simulink model "isubsystem_main"  (R2014b)
settings: Solver=ode45  StartTime=0.0  StopTime=5  FixedStep=0.001  RelTol=1e-3
undefined symbols (not defined in the file): v1, v10, v11, v12, v13, v14, v15, v16, v17, v18, v19, v2, v20, v21, v22, v3, v4, v5, v6, v7, v8, v9
(part 2 of 2)

== matlab function isubsystem_main/Subsystem/reduced-order dynamic gain observer/MATLAB Function ==
  data: lambda2 input; u input; dlambda2 output; yF input; k2 input; L input; dL input; x2_e output
function [dlambda2,x2_e]= fcn(lambda2,u,yF,k2,L,dL)
%#codegen

x2_e = lambda2 + k2*L*yF;
f1_yF = yF;f2_e = yF*x2_e;
dlambda2 = u + f2_e - k2*L*(x2_e + f1_yF)-k2*dL*yF;

== matlab function isubsystem_main/Subsystem/Fuzzy/MATLAB Function ==
  data: W input; yF input; Xi output; dW output; z1 input; Psi input; eta1 input
function [Xi,dW]= fcn(W,yF,z1,Psi,eta1)
%#codegen

Xi = [exp(-0.5*(yF - 8)^2);exp(-0.5*(yF - 4)^2);exp(-0.5*yF^2);exp(-0.5*(yF + 4)^2);exp(-0.5*(yF + 8)^2)];
dW = Psi*z1*Xi - eta1*Psi*W;

== matlab function isubsystem_main/Subsystem/reduced-order dynamic gain observer/Subsystem/MATLAB Function2 ==
  data: L input; yF input; dL output; sigma input; theta input; K input; P input; lP input; epsilon1 input; epsilon2 input; epsilon10 input; epsilon20 input; vartheta input
function dL = fcn(L,yF,sigma,theta,K,P,lP,epsilon1,epsilon2,epsilon10,epsilon20,vartheta)
%#codegen

hphou = 1 + 2*(yF)^2 + 2*(vartheta)^2;
a = (-theta + K)/sigma;
b = (norm(P,2)*epsilon1^2)/(lP*sigma) + ((2*epsilon10^2)^(-1)+(2*epsilon20^2)^(-1))/(lP*sigma);
c = (2*(2 + epsilon2^2)*norm(P,2)*(hphou)/(lP*sigma));
%dL = L/sigma*(-theta*L + norm(P,2)*epsilon1^2/lP + ((2*epsilon10^2)^(-1)+(2*epsilon20^2)^(-1))/lP + norm(P,2)*(epsilon2^4 + phou^2)/(lP*epsilon2^2) + K*L);
dL = a*L^2 + b*L + c*L;

== matlab function isubsystem_main/Subsystem/PPF /MATLAB Function ==
  data: psi0 input; psi output; dpsi output; psiinf input; T input; q input; t input; ddpsi output
function [psi,dpsi,ddpsi]= fcn(psi0,psiinf,T,q,t)
%#codegen
if t >= T
    r = 0;
    dr = 0;
    ddr = 0;
else
    r = (1 - T^(-1)*t)^(q+1)*(cos(3*t))^2;
    dr = -(cos(3*t)*(1 - t/T)^q*(cos(3*t) + q*cos(3*t) - 6*t*sin(3*t) + 6*T*sin(3*t)))/T;
    ddr = 18*sin(3*t)^2*(1 - t/T)^(q + 1) - 18*cos(3*t)^2*(1 - t/T)^(q + 1) + (q*cos(3*t)^2*(q + 1)*(1 - t/T)^(q - 1))/T^2 + (12*cos(3*t)*sin(3*t)*(q + 1)*(1 - t/T)^q)/T;
end
psi = (psi0 - psiinf)*r + psiinf;
dpsi = (psi0 - psiinf)*dr;
ddpsi = (psi0 - psiinf)*ddr;

== matlab function isubsystem_main/Subsystem/Controller1/Subsystem1/MATLAB Function2 ==
  data: dalpha1_dt input; dalpha1_dW input; dalpha1_dL input; dalpha1_dyF input; alpha1 input; yF input; lambda2 input; alpha2 output; dW input; dL input; L input; k2 input; gamma2 input; sigma input; epsilon20 input; epsilon11 input; epsilon22 input; epsilon23 input; epsilon24 input; epsilon25 input; z2 output
function [alpha2,z2] = fcn(dalpha1_dt,dalpha1_dW,dalpha1_dL,dalpha1_dyF,alpha1,yF,lambda2,dW,dL,L,k2,gamma2,sigma,epsilon20,epsilon11,epsilon22,epsilon23,epsilon24,epsilon25)
%#codegen

z2 = lambda2 - alpha1;
x2_e = lambda2 + k2*L*yF;
f1_yF = yF;f2_e = yF*x2_e;
alpha2 = f2_e - k2*L*(x2_e + f1_yF) - k2*dL*yF - dW'*dalpha1_dW - dalpha1_dL*dL - dalpha1_dt - dalpha1_dyF*(x2_e + f1_yF) + 0.5*z2*dalpha1_dyF^2*((epsilon20*L^sigma)^2 + epsilon22^2 + epsilon23^2 + epsilon25^2) + epsilon24^2*z2 + z2/(2*epsilon11^2) + gamma2*z2;

== matlab function isubsystem_main/Subsystem/Controller1/Subsystem2/MATLAB Function ==
  data: alpha2 input; v output; alpha1 input; lambda2 input; l1 input; l2 input; w input
function v = fcn(alpha2,alpha1,lambda2,l1,l2,w)
%#codegen
delta = 0.5;la = 1 - delta;
z2 = lambda2 - alpha1;
zetad = sqrt(z2^2*alpha2^2 + w^2);
%zetal = sqrt(z2^2*l2^2 + (1 - l1)^2*w^2);
zetal = sqrt(z2^2*l2^2 + w^2);
%v = -(1 + l1)*z2*(alpha2^2/zetad + l2^2/((1 - l1)*zetal));
v = -la^(-1)*z2*(alpha2^2/zetad + l2^2/(zetal));

== matlab function isubsystem_main/Subsystem/Controller1/Subsystem/MATLAB Function1 ==
  data: yF input; dalpha1_dt output; psi input; dpsi input; ddpsi input; L input; W input; Xi input; k2 input; b_low input; b_high input; li input; eta0 input; sigma input; gamma1 input; epsilon10 input; epsilon11 input; epsilon12 input; epsilon13 input; epsilon14 input; epsilon15 input; dalpha1_dW output; dalpha1_dL output; dalpha1_dyF output
function [dalpha1_dt,dalpha1_dW,dalpha1_dL,dalpha1_dyF]= fcn(yF,psi,dpsi,ddpsi,L,W,Xi,k2,b_low,b_high,li,eta0,sigma,gamma1,epsilon10,epsilon11,epsilon12,epsilon13,epsilon14,epsilon15)
%#codegen
dalpha1_dt = (yF*dpsi*(li^2 + yF^2)*(eta0 + 2*gamma1))/(2*li^2*psi^2) - (2*yF^3*dpsi*(b_high - yF/(psi*(li^2 + yF^2)^(1/2)))*(b_low + yF/(psi*(li^2 + yF^2)^(1/2)))*((li^4*(b_high*b_low + yF^2/(psi^2*(li^2 + yF^2)))^2*(epsilon11^2 + epsilon12^2 + epsilon13^2 + epsilon15^2))/(2*(li^2 + yF^2)^3*(b_high - yF/(psi*(li^2 + yF^2)^(1/2)))^4*(b_low + yF/(psi*(li^2 + yF^2)^(1/2)))^4) + (L^(2*sigma)*epsilon10^2*li^4*(b_high*b_low + yF^2/(psi^2*(li^2 + yF^2)))^2)/(2*(li^2 + yF^2)^3*(b_high - yF/(psi*(li^2 + yF^2)^(1/2)))^4*(b_low + yF/(psi*(li^2 + yF^2)^(1/2)))^4) + (epsilon14^2*yF^2*dpsi^2*(b_high*b_low + yF^2/(psi^2*(li^2 + yF^2)))^2)/(2*psi^4*(li^2 + yF^2)*(b_high - yF/(psi*(li^2 + yF^2)^(1/2)))^4*(b_low + yF/(psi*(li^2 + yF^2)^(1/2)))^4)))/(li^2*psi^4*(b_high*b_low + yF^2/(psi^2*(li^2 + yF^2)))^2) + (yF*(li^2 + yF^2)*(b_high - yF/(psi*(li^2 + yF^2)^(1/2)))*(b_low + yF/(psi*(li^2 + yF^2)^(1/2)))*((2*epsilon14^2*yF^2*dpsi*dpsi^2*(b_high*b_low + yF^2/(psi^2*(li^2 + yF^2)))^2)/(psi^5*(li^2 + yF^2)*(b_high - yF/(psi*(li^2 + yF^2)^(1/2)))^4*(b_low + yF/(psi*(li^2 + yF^2)^(1/2)))^4) - (2*epsilon14^2*yF^3*dpsi*dpsi^2*(b_high*b_low + yF^2/(psi^2*(li^2 + yF^2)))^2)/(psi^6*(li^2 + yF^2)^(3/2)*(b_high - yF/(psi*(li^2 + yF^2)^(1/2)))^4*(b_low + yF/(psi*(li^2 + yF^2)^(1/2)))^5) + (2*epsilon14^2*yF^3*dpsi*dpsi^2*(b_high*b_low + yF^2/(psi^2*(li^2 + yF^2)))^2)/(psi^6*(li^2 + yF^2)^(3/2)*(b_high - yF/(psi*(li^2 + yF^2)^(1/2)))^5*(b_low + yF/(psi*(li^2 + yF^2)^(1/2)))^4) - (epsilon14^2*yF^2*ddpsi*dpsi*(b_high*b_low + yF^2/(psi^2*(li^2 + yF^2)))^2)/(psi^4*(li^2 + yF^2)*(b_high - yF/(psi*(li^2 + yF^2)^(1/2)))^4*(b_low + yF/(psi*(li^2 + yF^2)^(1/2)))^4) + (2*epsilon14^2*yF^4*dpsi*dpsi^2*(b_high*b_low + yF^2/(psi^2*(li^2 + yF^2))))/(psi^7*(li^2 + yF^2)^2*(b_high - yF/(psi*(li^2 + yF^2)^(1/2)))^4*(b_low + yF/(psi*(li^2 + yF^2)^(1/2)))^4) + (2*li^4*yF^2*dpsi*(b_high*b_low + yF^2/(psi^2*(li^2 + yF^2)))*(epsilon11^2 + epsilon12^2 + epsilon13^2 + epsilon15^2))/(psi^3*(li^2 + yF^2)^4*(b_high - yF/(psi*(li^2 + yF^2)^(1/2)))^4*(b_low + yF/(psi*(li^2 + yF^2)^(1/2)))^4) - (2*li^4*yF*dpsi*(b_high*b_low + yF^2/(psi^2*(li^2 + yF^2)))^2*(epsilon11^2 + epsilon12^2 + epsilon13^2 + epsilon15^2))/(psi^2*(li^2 + yF^2)^(7/2)*(b_high - yF/(psi*(li^2 + yF^2)^(1/2)))^4*(b_low + yF/(psi*(li^2 + yF^2)^(1/2)))^5) + (2*li^4*yF*dpsi*(b_high*b_low + yF^2/(psi^2*(li^2 + yF^2)))^2*(epsilon11^2 + epsilon12^2 + epsilon13^2 + epsilon15^2))/(psi^2*(li^2 + yF^2)^(7/2)*(b_high - yF/(psi*(li^2 + yF^2)^(1/2)))^5*(b_low + yF/(psi*(li^2 + yF^2)^(1/2)))^4) + (2*L^(2*sigma)*epsilon10^2*li^4*yF^2*dpsi*(b_high*b_low + yF^2/(psi^2*(li^2 + yF^2))))/(psi^3*(li^2 + yF^2)^4*(b_high - yF/(psi*(li^2 + yF^2)^(1/2)))^4*(b_low + yF/(psi*(li^2 + yF^2)^(1/2)))^4) - (2*L^(2*sigma)*epsilon10^2*li^4*yF*dpsi*(b_high*b_low + yF^2/(psi^2*(li^2 + yF^2)))^2)/(psi^2*(li^2 + yF^2)^(7/2)*(b_high - yF/(psi*(li^2 + yF^2)^(1/2)))^4*(b_low + yF/(psi*(li^2 + yF^2)^(1/2)))^5) + (2*L^(2*sigma)*epsilon10^2*li^4*yF*dpsi*(b_high*b_low + yF^2/(psi^2*(li^2 + yF^2)))^2)/(psi^2*(li^2 + yF^2)^(7/2)*(b_high - yF/(psi*(li^2 + yF^2)^(1/2)))^5*(b_low + yF/(psi*(li^2 + yF^2)^(1/2)))^4)))/(li^2*psi*(b_high*b_low + yF^2/(psi^2*(li^2 + yF^2)))) + (yF^2*dpsi*(li^2 + yF^2)^(1/2)*(b_high - yF/(psi*(li^2 + yF^2)^(1/2)))*((li^4*(b_high*b_low + yF^2/(psi^2*(li^2 + yF^2)))^2*(epsilon11^2 + epsilon12^2 + epsilon13^2 + epsilon15^2))/(2*(li^2 + yF^2)^3*(b_high - yF/(psi*(li^2 + yF^2)^(1/2)))^4*(b_low + yF/(psi*(li^2 + yF^2)^(1/2)))^4) + (L^(2*sigma)*epsilon10^2*li^4*(b_high*b_low + yF^2/(psi^2*(li^2 + yF^2)))^2)/(2*(li^2 + yF^2)^3*(b_high - yF/(psi*(li^2 + yF^2)^(1/2)))^4*(b_low + yF/(psi*(li^2 + yF^2)^(1/2)))^4) + (epsilon14^2*yF^2*dpsi^2*(b_high*b_low + yF^2/(psi^2*(li^2 + yF^2)))^2)/(2*psi^4*(li^2 + yF^2)*(b_high - yF/(psi*(li^2 + yF^2)^(1/2)))^4*(b_low + yF/(psi*(li^2 + yF^2)^(1/2)))^4)))/(li^2*psi^3*(b_high*b_low + yF^2/(psi^2*(li^2 + yF^2)))) - (yF^2*dpsi*(li^2 + yF^2)^(1/2)*(b_low + yF/(psi*(li^2 + yF^2)^(1/2)))*((li^4*(b_high*b_low + yF^2/(psi^2*(li^2 + yF^2)))^2*(epsilon11^2 + epsilon12^2 + epsilon13^2 + epsilon15^2))/(2*(li^2 + yF^2)^3*(b_high - yF/(psi*(li^2 + yF^2)^(1/2)))^4*(b_low + yF/(psi*(li^2 + yF^2)^(1/2)))^4) + (L^(2*sigma)*epsilon10^2*li^4*(b_high*b_low + yF^2/(psi^2*(li^2 + yF^2)))^2)/(2*(li^2 + yF^2)^3*(b_high - yF/(psi*(li^2 + yF^2)^(1/2)))^4*(b_low + yF/(psi*(li^2 + yF^2)^(1/2)))^4) + (epsilon14^2*yF^2*dpsi^2*(b_high*b_low + yF^2/(psi^2*(li^2 + yF^2)))^2)/(2*psi^4*(li^2 + yF^2)*(b_high - yF/(psi*(li^2 + yF^2)^(1/2)))^4*(b_low + yF/(psi*(li^2 + yF^2)^(1/2)))^4)))/(li^2*psi^3*(b_high*b_low + yF^2/(psi^2*(li^2 + yF^2)))) + (yF*dpsi*(li^2 + yF^2)*(b_high - yF/(psi*(li^2 + yF^2)^(1/2)))*(b_low + yF/(psi*(li^2 + yF^2)^(1/2)))*((li^4*(b_high*b_low + yF^2/(psi^2*(li^2 + yF^2)))^2*(epsilon11^2 + epsilon12^2 + epsilon13^2 + epsilon15^2))/(2*(li^2 + yF^2)^3*(b_high - yF/(psi*(li^2 + yF^2)^(1/2)))^4*(b_low + yF/(psi*(li^2 + yF^2)^(1/2)))^4) + (L^(2*sigma)*epsilon10^2*li^4*(b_high*b_low + yF^2/(psi^2*(li^2 + yF^2)))^2)/(2*(li^2 + yF^2)^3*(b_high - yF/(psi*(li^2 + yF^2)^(1/2)))^4*(b_low + yF/(psi*(li^2 + yF^2)^(1/2)))^4) + (epsilon14^2*yF^2*dpsi^2*(b_high*b_low + yF^2/(psi^2*(li^2 + yF^2)))^2)/(2*psi^4*(li^2 + yF^2)*(b_high - yF/(psi*(li^2 + yF^2)^(1/2)))^4*(b_low + yF/(psi*(li^2 + yF^2)^(1/2)))^4)))/(li^2*psi^2*(b_high*b_low + yF^2/(psi^2*(li^2 + yF^2)))) - (yF*dpsi*(li^2 + yF^2)*(b_high - yF/(psi*(li^2 + yF^2)^(1/2)))*(b_low + yF/(psi*(li^2 + yF^2)^(1/2)))^2*(eta0*yF*psi*(li^2 + yF^2)^(1/2) - 2*W'*Xi*yF^2 + 2*gamma1*yF*psi*(li^2 + yF^2)^(1/2) + 2*W'*Xi*b_high*yF*psi*(li^2 + yF^2)^(1/2) - 2*W'*Xi*b_low*yF*psi*(li^2 + yF^2)^(1/2) + 2*W'*Xi*b_high*b_low*li^2*psi^2 + 2*W'*Xi*b_high*b_low*yF^2*psi^2))/(li^2*psi^2*(b_high*b_low + yF^2/(psi^2*(li^2 + yF^2)))*(b_high*b_low*li^2*psi^2 - yF^2 + b_high*b_low*yF^2*psi^2 + b_high*yF*psi*(li^2 + yF^2)^(1/2) - b_low*yF*psi*(li^2 + yF^2)^(1/2))) + (yF*dpsi*(li^2 + yF^2)*(b_high - yF/(psi*(li^2 + yF^2)^(1/2)))^2*(b_low + yF/(psi*(li^2 + yF^2)^(1/2)))*(eta0*yF*psi*(li^2 + yF^2)^(1/2) - 2*W'*Xi*yF^2 + 2*gamma1*yF*psi*(li^2 + yF^2)^(1/2) + 2*W'*Xi*b_high*yF*psi*(li^2 + yF^2)^(1/2) - 2*W'*Xi*b_low*yF*psi*(li^2 + yF^2)^(1/2) + 2*W'*Xi*b_high*b_low*li^2*psi^2 + 2*W'*Xi*b_high*b_low*yF^2*psi^2))/(li^2*psi^2*(b_high*b_low + yF^2/(psi^2*(li^2 + yF^2)))*(b_high*b_low*li^2*psi^2 - yF^2 + b_high*b_low*yF^2*psi^2 + b_high*yF*psi*(li^2 + yF^2)^(1/2) - b_low*yF*psi*(li^2 + yF^2)^(1/2))) - (yF^2*dpsi*(li^2 + yF^2)^(1/2)*(b_high - yF/(psi*(li^2 + yF^2)^(1/2)))^2*(b_low + yF/(psi*(li^2 + yF^2)^(1/2)))^2*(eta0*yF*psi*(li^2 + yF^2)^(1/2) - 2*W'*Xi*yF^2 + 2*gamma1*yF*psi*(li^2 + yF^2)^(1/2) + 2*W'*Xi*b_high*yF*psi*(li^2 + yF^2)^(1/2) - 2*W'*Xi*b_low*yF*psi*(li^2 + yF^2)^(1/2) + 2*W'*Xi*b_high*b_low*li^2*psi^2 + 2*W'*Xi*b_high*b_low*yF^2*psi^2))/(li^2*psi^3*(b_high*b_low + yF^2/(psi^2*(li^2 + yF^2)))^2*(b_high*b_low*li^2*psi^2 - yF^2 + b_high*b_low*yF^2*psi^2 + b_high*yF*psi*(li^2 + yF^2)^(1/2) - b_low*yF*psi*(li^2 + yF^2)^(1/2)));
dalpha1_dW = -(Xi*(li^2 + yF^2)^(3/2)*(b_high - yF/(psi*(li^2 + yF^2)^(1/2)))^2*(b_low + yF/(psi*(li^2 + yF^2)^(1/2)))^2)/(li^2*(b_high*b_low + yF^2/(psi^2*(li^2 + yF^2)))); 
dalpha1_dL = - k2*yF - (L^(2*sigma - 1)*epsilon10^2*li^2*sigma*yF*(b_high*b_low + yF^2/(psi^2*(li^2 + yF^2))))/(psi*(li^2 + yF^2)^2*(b_high - yF/(psi*(li^2 + yF^2)^(1/2)))^3*(b_low + yF/(psi*(li^2 + yF^2)^(1/2)))^3);
dalpha1_dyF = (b_high - yF/(psi*(li^2 + yF^2)^(1/2)))*(b_low + yF/(psi*(li^2 + yF^2)^(1/2)))^2*(eta0*yF*psi*(li^2 + yF^2)^(1/2) - 2*W'*Xi*yF^2 + 2*gamma1*yF*psi*(li^2 + yF^2)^(1/2) + 2*W'*Xi*b_high*yF*psi*(li^2 + yF^2)^(1/2) - 2*W'*Xi*b_low*yF*psi*(li^2 + yF^2)^(1/2) + 2*W'*Xi*b_high*b_low*li^2*psi^2 + 2*W'*Xi*b_high*b_low*yF^2*psi^2);

== matlab function isubsystem_main/Subsystem/Controller1/Subsystem3/MATLAB Function1 ==
  data: yF input; alpha1 output; psi input; dpsi input; L input; W input; Xi input; k2 input; b_low input; b_high input; li input; eta0 input; sigma input; gamma1 input; epsilon10 input; epsilon11 input; epsilon12 input; epsilon13 input; epsilon14 input; epsilon15 input; z1 output
function [alpha1,z1]= fcn(yF,psi,dpsi,L,W,Xi,k2,b_low,b_high,li,eta0,sigma,gamma1,epsilon10,epsilon11,epsilon12,epsilon13,epsilon14,epsilon15)
%#codegen
f1_yF = yF;
X = yF/(psi*sqrt(yF^2 + li^2));
z1 = X/((b_low + X)*(b_high - X));
h1 = li^2*(b_low*b_high + X^2)/((b_low+X)^2*(b_high-X)^2*(yF^2 + li^2)^(3/2));
h2 = -dpsi*yF*(b_low*b_high + X^2)/(psi^2*(b_low+X)^2*(b_high-X)^2*sqrt(yF^2 + li^2));
alpha1 = - k2*L*yF - f1_yF - h1^(-1)*(W'*Xi + gamma1*z1 + eta0/2*z1)-z1*h1^(-1)*(0.5*(epsilon10*h1*L^sigma)^2 + 0.5*h1^2*(epsilon11^2 + epsilon12^2 + epsilon13^2 + epsilon15^2) + 0.5*(epsilon14*h2)^2);

== matlab function isubsystem_main/Event-Triggered/MATLAB Function ==
  data: miu input; E_out output; miu_tk input; eta output; triger output
function [E_out,eta, triger]= fcn(miu,miu_tk)
%#codegen
E_miu = miu_tk;
eta = miu - E_miu;
l1 = 0.2;l2 = 1.5;
triger = (abs(eta)>= l1*abs(E_miu)+l2).*1;
if abs(eta)>= l1*abs(E_miu)+l2
    E_out = miu;
else
    E_out = miu_tk;
end

== matlab function isubsystem_main/Hysteretic Quantizer/MATLAB Function ==
  data: miu input; Q_miu output; Output_t input; dmiu input
function Q_miu = fcn(miu,Output_t,dmiu)
%#codegen
i = (1:1:100)';
delta = 0.5;miu_min = 0.05;
la = 1 - delta;lb = 1 + delta;lc = la/lb;
miu_i = lc.^(1-i).*miu_min;

if dmiu < 0
    A = (((abs(miu)<=(miu_i/la))*1).*((abs(miu)>(miu_i/lb))*1))';
    miui = A*miu_i;
    if abs(miu) >= 0 && abs(miu) < miu_min/lb
        Output = 0;
    else
        if abs(miu) <= miui && abs(miu) > miui/lb
            Output = miui*sign(miu);
        else
            Output = miui*lb*sign(miu);
        end
    end
elseif dmiu > 0
    A = (((abs(miu)<=(miu_i*lb/la))*1).*((abs(miu)>(miu_i))*1))';
    miui = A*miu_i;
    if abs(miu) >= miu_min/lb && abs(miu) < miu_min
        Output = 0;
    else
        if abs(miu) <= miui/la && abs(miu) > miui
            Output = miui*sign(miu);
        else
            Output = miui*lb*sign(miu);
        end
    end
else
    Output = Output_t;
end

Q_miu = Output;

== matlab function isubsystem_main/Subsystem1/Controller1/Subsystem/MATLAB Function1 ==
  data: yF input; dalpha1_dt output; psi input; dpsi input; ddpsi input; L input; W input; Xi input; k2 input; b_low input; b_high input; li input; eta0 input; sigma input; gamma1 input; epsilon10 input; epsilon11 input; epsilon12 input; epsilon13 input; epsilon14 input; epsilon15 input; dalpha1_dW output; dalpha1_dL output; dalpha1_dyF output
function [dalpha1_dt,dalpha1_dW,dalpha1_dL,dalpha1_dyF]= fcn(yF,psi,dpsi,ddpsi,L,W,Xi,k2,b_low,b_high,li,eta0,sigma,gamma1,epsilon10,epsilon11,epsilon12,epsilon13,epsilon14,epsilon15)
%#codegen
dalpha1_dt = (yF*dpsi*(li^2 + yF^2)*(eta0 + 2*gamma1))/(2*li^2*psi^2) - (2*yF^3*dpsi*(b_high - yF/(psi*(li^2 + yF^2)^(1/2)))*(b_low + yF/(psi*(li^2 + yF^2)^(1/2)))*((li^4*(b_high*b_low + yF^2/(psi^2*(li^2 + yF^2)))^2*(epsilon11^2 + epsilon12^2 + epsilon13^2 + epsilon15^2))/(2*(li^2 + yF^2)^3*(b_high - yF/(psi*(li^2 + yF^2)^(1/2)))^4*(b_low + yF/(psi*(li^2 + yF^2)^(1/2)))^4) + (L^(2*sigma)*epsilon10^2*li^4*(b_high*b_low + yF^2/(psi^2*(li^2 + yF^2)))^2)/(2*(li^2 + yF^2)^3*(b_high - yF/(psi*(li^2 + yF^2)^(1/2)))^4*(b_low + yF/(psi*(li^2 + yF^2)^(1/2)))^4) + (epsilon14^2*yF^2*dpsi^2*(b_high*b_low + yF^2/(psi^2*(li^2 + yF^2)))^2)/(2*psi^4*(li^2 + yF^2)*(b_high - yF/(psi*(li^2 + yF^2)^(1/2)))^4*(b_low + yF/(psi*(li^2 + yF^2)^(1/2)))^4)))/(li^2*psi^4*(b_high*b_low + yF^2/(psi^2*(li^2 + yF^2)))^2) + (yF*(li^2 + yF^2)*(b_high - yF/(psi*(li^2 + yF^2)^(1/2)))*(b_low + yF/(psi*(li^2 + yF^2)^(1/2)))*((2*epsilon14^2*yF^2*dpsi*dpsi^2*(b_high*b_low + yF^2/(psi^2*(li^2 + yF^2)))^2)/(psi^5*(li^2 + yF^2)*(b_high - yF/(psi*(li^2 + yF^2)^(1/2)))^4*(b_low + yF/(psi*(li^2 + yF^2)^(1/2)))^4) - (2*epsilon14^2*yF^3*dpsi*dpsi^2*(b_high*b_low + yF^2/(psi^2*(li^2 + yF^2)))^2)/(psi^6*(li^2 + yF^2)^(3/2)*(b_high - yF/(psi*(li^2 + yF^2)^(1/2)))^4*(b_low + yF/(psi*(li^2 + yF^2)^(1/2)))^5) + (2*epsilon14^2*yF^3*dpsi*dpsi^2*(b_high*b_low + yF^2/(psi^2*(li^2 + yF^2)))^2)/(psi^6*(li^2 + yF^2)^(3/2)*(b_high - yF/(psi*(li^2 + yF^2)^(1/2)))^5*(b_low + yF/(psi*(li^2 + yF^2)^(1/2)))^4) - (epsilon14^2*yF^2*ddpsi*dpsi*(b_high*b_low + yF^2/(psi^2*(li^2 + yF^2)))^2)/(psi^4*(li^2 + yF^2)*(b_high - yF/(psi*(li^2 + yF^2)^(1/2)))^4*(b_low + yF/(psi*(li^2 + yF^2)^(1/2)))^4) + (2*epsilon14^2*yF^4*dpsi*dpsi^2*(b_high*b_low + yF^2/(psi^2*(li^2 + yF^2))))/(psi^7*(li^2 + yF^2)^2*(b_high - yF/(psi*(li^2 + yF^2)^(1/2)))^4*(b_low + yF/(psi*(li^2 + yF^2)^(1/2)))^4) + (2*li^4*yF^2*dpsi*(b_high*b_low + yF^2/(psi^2*(li^2 + yF^2)))*(epsilon11^2 + epsilon12^2 + epsilon13^2 + epsilon15^2))/(psi^3*(li^2 + yF^2)^4*(b_high - yF/(psi*(li^2 + yF^2)^(1/2)))^4*(b_low + yF/(psi*(li^2 + yF^2)^(1/2)))^4) - (2*li^4*yF*dpsi*(b_high*b_low + yF^2/(psi^2*(li^2 + yF^2)))^2*(epsilon11^2 + epsilon12^2 + epsilon13^2 + epsilon15^2))/(psi^2*(li^2 + yF^2)^(7/2)*(b_high - yF/(psi*(li^2 + yF^2)^(1/2)))^4*(b_low + yF/(psi*(li^2 + yF^2)^(1/2)))^5) + (2*li^4*yF*dpsi*(b_high*b_low + yF^2/(psi^2*(li^2 + yF^2)))^2*(epsilon11^2 + epsilon12^2 + epsilon13^2 + epsilon15^2))/(psi^2*(li^2 + yF^2)^(7/2)*(b_high - yF/(psi*(li^2 + yF^2)^(1/2)))^5*(b_low + yF/(psi*(li^2 + yF^2)^(1/2)))^4) + (2*L^(2*sigma)*epsilon10^2*li^4*yF^2*dpsi*(b_high*b_low + yF^2/(psi^2*(li^2 + yF^2))))/(psi^3*(li^2 + yF^2)^4*(b_high - yF/(psi*(li^2 + yF^2)^(1/2)))^4*(b_low + yF/(psi*(li^2 + yF^2)^(1/2)))^4) - (2*L^(2*sigma)*epsilon10^2*li^4*yF*dpsi*(b_high*b_low + yF^2/(psi^2*(li^2 + yF^2)))^2)/(psi^2*(li^2 + yF^2)^(7/2)*(b_high - yF/(psi*(li^2 + yF^2)^(1/2)))^4*(b_low + yF/(psi*(li^2 + yF^2)^(1/2)))^5) + (2*L^(2*sigma)*epsilon10^2*li^4*yF*dpsi*(b_high*b_low + yF^2/(psi^2*(li^2 + yF^2)))^2)/(psi^2*(li^2 + yF^2)^(7/2)*(b_high - yF/(psi*(li^2 + yF^2)^(1/2)))^5*(b_low + yF/(psi*(li^2 + yF^2)^(1/2)))^4)))/(li^2*psi*(b_high*b_low + yF^2/(psi^2*(li^2 + yF^2)))) + (yF^2*dpsi*(li^2 + yF^2)^(1/2)*(b_high - yF/(psi*(li^2 + yF^2)^(1/2)))*((li^4*(b_high*b_low + yF^2/(psi^2*(li^2 + yF^2)))^2*(epsilon11^2 + epsilon12^2 + epsilon13^2 + epsilon15^2))/(2*(li^2 + yF^2)^3*(b_high - yF/(psi*(li^2 + yF^2)^(1/2)))^4*(b_low + yF/(psi*(li^2 + yF^2)^(1/2)))^4) + (L^(2*sigma)*epsilon10^2*li^4*(b_high*b_low + yF^2/(psi^2*(li^2 + yF^2)))^2)/(2*(li^2 + yF^2)^3*(b_high - yF/(psi*(li^2 + yF^2)^(1/2)))^4*(b_low + yF/(psi*(li^2 + yF^2)^(1/2)))^4) + (epsilon14^2*yF^2*dpsi^2*(b_high*b_low + yF^2/(psi^2*(li^2 + yF^2)))^2)/(2*psi^4*(li^2 + yF^2)*(b_high - yF/(psi*(li^2 + yF^2)^(1/2)))^4*(b_low + yF/(psi*(li^2 + yF^2)^(1/2)))^4)))/(li^2*psi^3*(b_high*b_low + yF^2/(psi^2*(li^2 + yF^2)))) - (yF^2*dpsi*(li^2 + yF^2)^(1/2)*(b_low + yF/(psi*(li^2 + yF^2)^(1/2)))*((li^4*(b_high*b_low + yF^2/(psi^2*(li^2 + yF^2)))^2*(epsilon11^2 + epsilon12^2 + epsilon13^2 + epsilon15^2))/(2*(li^2 + yF^2)^3*(b_high - yF/(psi*(li^2 + yF^2)^(1/2)))^4*(b_low + yF/(psi*(li^2 + yF^2)^(1/2)))^4) + (L^(2*sigma)*epsilon10^2*li^4*(b_high*b_low + yF^2/(psi^2*(li^2 + yF^2)))^2)/(2*(li^2 + yF^2)^3*(b_high - yF/(psi*(li^2 + yF^2)^(1/2)))^4*(b_low + yF/(psi*(li^2 + yF^2)^(1/2)))^4) + (epsilon14^2*yF^2*dpsi^2*(b_high*b_low + yF^2/(psi^2*(li^2 + yF^2)))^2)/(2*psi^4*(li^2 + yF^2)*(b_high - yF/(psi*(li^2 + yF^2)^(1/2)))^4*(b_low + yF/(psi*(li^2 + yF^2)^(1/2)))^4)))/(li^2*psi^3*(b_high*b_low + yF^2/(psi^2*(li^2 + yF^2)))) + (yF*dpsi*(li^2 + yF^2)*(b_high - yF/(psi*(li^2 + yF^2)^(1/2)))*(b_low + yF/(psi*(li^2 + yF^2)^(1/2)))*((li^4*(b_high*b_low + yF^2/(psi^2*(li^2 + yF^2)))^2*(epsilon11^2 + epsilon12^2 + epsilon13^2 + epsilon15^2))/(2*(li^2 + yF^2)^3*(b_high - yF/(psi*(li^2 + yF^2)^(1/2)))^4*(b_low + yF/(psi*(li^2 + yF^2)^(1/2)))^4) + (L^(2*sigma)*epsilon10^2*li^4*(b_high*b_low + yF^2/(psi^2*(li^2 + yF^2)))^2)/(2*(li^2 + yF^2)^3*(b_high - yF/(psi*(li^2 + yF^2)^(1/2)))^4*(b_low + yF/(psi*(li^2 + yF^2)^(1/2)))^4) + (epsilon14^2*yF^2*dpsi^2*(b_high*b_low + yF^2/(psi^2*(li^2 + yF^2)))^2)/(2*psi^4*(li^2 + yF^2)*(b_high - yF/(psi*(li^2 + yF^2)^(1/2)))^4*(b_low + yF/(psi*(li^2 + yF^2)^(1/2)))^4)))/(li^2*psi^2*(b_high*b_low + yF^2/(psi^2*(li^2 + yF^2)))) - (yF*dpsi*(li^2 + yF^2)*(b_high - yF/(psi*(li^2 + yF^2)^(1/2)))*(b_low + yF/(psi*(li^2 + yF^2)^(1/2)))^2*(eta0*yF*psi*(li^2 + yF^2)^(1/2) - 2*W'*Xi*yF^2 + 2*gamma1*yF*psi*(li^2 + yF^2)^(1/2) + 2*W'*Xi*b_high*yF*psi*(li^2 + yF^2)^(1/2) - 2*W'*Xi*b_low*yF*psi*(li^2 + yF^2)^(1/2) + 2*W'*Xi*b_high*b_low*li^2*psi^2 + 2*W'*Xi*b_high*b_low*yF^2*psi^2))/(li^2*psi^2*(b_high*b_low + yF^2/(psi^2*(li^2 + yF^2)))*(b_high*b_low*li^2*psi^2 - yF^2 + b_high*b_low*yF^2*psi^2 + b_high*yF*psi*(li^2 + yF^2)^(1/2) - b_low*yF*psi*(li^2 + yF^2)^(1/2))) + (yF*dpsi*(li^2 + yF^2)*(b_high - yF/(psi*(li^2 + yF^2)^(1/2)))^2*(b_low + yF/(psi*(li^2 + yF^2)^(1/2)))*(eta0*yF*psi*(li^2 + yF^2)^(1/2) - 2*W'*Xi*yF^2 + 2*gamma1*yF*psi*(li^2 + yF^2)^(1/2) + 2*W'*Xi*b_high*yF*psi*(li^2 + yF^2)^(1/2) - 2*W'*Xi*b_low*yF*psi*(li^2 + yF^2)^(1/2) + 2*W'*Xi*b_high*b_low*li^2*psi^2 + 2*W'*Xi*b_high*b_low*yF^2*psi^2))/(li^2*psi^2*(b_high*b_low + yF^2/(psi^2*(li^2 + yF^2)))*(b_high*b_low*li^2*psi^2 - yF^2 + b_high*b_low*yF^2*psi^2 + b_high*yF*psi*(li^2 + yF^2)^(1/2) - b_low*yF*psi*(li^2 + yF^2)^(1/2))) - (yF^2*dpsi*(li^2 + yF^2)^(1/2)*(b_high - yF/(psi*(li^2 + yF^2)^(1/2)))^2*(b_low + yF/(psi*(li^2 + yF^2)^(1/2)))^2*(eta0*yF*psi*(li^2 + yF^2)^(1/2) - 2*W'*Xi*yF^2 + 2*gamma1*yF*psi*(li^2 + yF^2)^(1/2) + 2*W'*Xi*b_high*yF*psi*(li^2 + yF^2)^(1/2) - 2*W'*Xi*b_low*yF*psi*(li^2 + yF^2)^(1/2) + 2*W'*Xi*b_high*b_low*li^2*psi^2 + 2*W'*Xi*b_high*b_low*yF^2*psi^2))/(li^2*psi^3*(b_high*b_low + yF^2/(psi^2*(li^2 + yF^2)))^2*(b_high*b_low*li^2*psi^2 - yF^2 + b_high*b_low*yF^2*psi^2 + b_high*yF*psi*(li^2 + yF^2)^(1/2) - b_low*yF*psi*(li^2 + yF^2)^(1/2)));
dalpha1_dW = -(Xi*(li^2 + yF^2)^(3/2)*(b_high - yF/(psi*(li^2 + yF^2)^(1/2)))^2*(b_low + yF/(psi*(li^2 + yF^2)^(1/2)))^2)/(li^2*(b_high*b_low + yF^2/(psi^2*(li^2 + yF^2)))); 
dalpha1_dL = - k2*yF - (L^(2*sigma - 1)*epsilon10^2*li^2*sigma*yF*(b_high*b_low + yF^2/(psi^2*(li^2 + yF^2))))/(psi*(li^2 + yF^2)^2*(b_high - yF/(psi*(li^2 + yF^2)^(1/2)))^3*(b_low + yF/(psi*(li^2 + yF^2)^(1/2)))^3);
dalpha1_dyF = (b_high - yF/(psi*(li^2 + yF^2)^(1/2)))*(b_low + yF/(psi*(li^2 + yF^2)^(1/2)))^2*(eta0*yF*psi*(li^2 + yF^2)^(1/2) - 2*W'*Xi*yF^2 + 2*gamma1*yF*psi*(li^2 + yF^2)^(1/2) + 2*W'*Xi*b_high*yF*psi*(li^2 + yF^2)^(1/2) - 2*W'*Xi*b_low*yF*psi*(li^2 + yF^2)^(1/2) + 2*W'*Xi*b_high*b_low*li^2*psi^2 + 2*W'*Xi*b_high*b_low*yF^2*psi^2);

== matlab function isubsystem_main/Subsystem1/Controller1/Subsystem1/MATLAB Function2 ==
  data: dalpha1_dt input; dalpha1_dW input; dalpha1_dL input; dalpha1_dyF input; alpha1 input; yF input; lambda2 input; alpha2 output; dW input; dL input; L input; k2 input; gamma2 input; sigma input; epsilon20 input; epsilon11 input; epsilon22 input; epsilon23 input; epsilon24 input; epsilon25 input; z2 output
function [alpha2,z2] = fcn(dalpha1_dt,dalpha1_dW,dalpha1_dL,dalpha1_dyF,alpha1,yF,lambda2,dW,dL,L,k2,gamma2,sigma,epsilon20,epsilon11,epsilon22,epsilon23,epsilon24,epsilon25)
%#codegen

z2 = lambda2 - alpha1;
x2_e = lambda2 + k2*L*yF;
f1_yF = yF;f2_e = yF*x2_e;
alpha2 = f2_e - k2*L*(x2_e + f1_yF) - k2*dL*yF - dW'*dalpha1_dW - dalpha1_dL*dL - dalpha1_dt - dalpha1_dyF*(x2_e + f1_yF) + 0.5*z2*dalpha1_dyF^2*((epsilon20*L^sigma)^2 + epsilon22^2 + epsilon23^2 + epsilon25^2) + epsilon24^2*z2 + z2/(2*epsilon11^2) + gamma2*z2;

== matlab function isubsystem_main/Subsystem1/Controller1/Subsystem2/MATLAB Function ==
  data: alpha2 input; v output; alpha1 input; lambda2 input; l1 input; l2 input; w input
function v = fcn(alpha2,alpha1,lambda2,l1,l2,w)
%#codegen
delta = 0.5;la = 1 - delta;
z2 = lambda2 - alpha1;
zetad = sqrt(z2^2*alpha2^2 + w^2);
%zetal = sqrt(z2^2*l2^2 + (1 - l1)^2*w^2);
zetal = sqrt(z2^2*l2^2 + w^2);
%v = -(1 + l1)*z2*(alpha2^2/zetad + l2^2/((1 - l1)*zetal));
v = -la^(-1)*z2*(alpha2^2/zetad + l2^2/(zetal));

== matlab function isubsystem_main/Subsystem1/Controller1/Subsystem3/MATLAB Function1 ==
  data: yF input; alpha1 output; psi input; dpsi input; L input; W input; Xi input; k2 input; b_low input; b_high input; li input; eta0 input; sigma input; gamma1 input; epsilon10 input; epsilon11 input; epsilon12 input; epsilon13 input; epsilon14 input; epsilon15 input; z1 output
function [alpha1,z1]= fcn(yF,psi,dpsi,L,W,Xi,k2,b_low,b_high,li,eta0,sigma,gamma1,epsilon10,epsilon11,epsilon12,epsilon13,epsilon14,epsilon15)
%#codegen
f1_yF = yF;
X = yF/(psi*sqrt(yF^2 + li^2));
z1 = X/((b_low + X)*(b_high - X));
h1 = li^2*(b_low*b_high + X^2)/((b_low+X)^2*(b_high-X)^2*(yF^2 + li^2)^(3/2));
h2 = -dpsi*yF*(b_low*b_high + X^2)/(psi^2*(b_low+X)^2*(b_high-X)^2*sqrt(yF^2 + li^2));
alpha1 = - k2*L*yF - f1_yF - h1^(-1)*(W'*Xi + gamma1*z1 + eta0/2*z1)-z1*h1^(-1)*(0.5*(epsilon10*h1*L^sigma)^2 + 0.5*h1^2*(epsilon11^2 + epsilon12^2 + epsilon13^2 + epsilon15^2) + 0.5*(epsilon14*h2)^2);

== matlab function isubsystem_main/Subsystem1/Fuzzy/MATLAB Function ==
  data: W input; yF input; Xi output; dW output; z1 input; Psi input; eta1 input
function [Xi,dW]= fcn(W,yF,z1,Psi,eta1)
%#codegen

Xi = [exp(-0.5*(yF - 8)^2);exp(-0.5*(yF - 4)^2);exp(-0.5*yF^2);exp(-0.5*(yF + 4)^2);exp(-0.5*(yF + 8)^2)];
dW = Psi*z1*Xi - eta1*Psi*W;

== matlab function isubsystem_main/Subsystem1/PPF /MATLAB Function ==
  data: psi0 input; psi output; dpsi output; psiinf input; T input; q input; t input; ddpsi output
function [psi,dpsi,ddpsi]= fcn(psi0,psiinf,T,q,t)
%#codegen
if t >= T
    r = 0;
    dr = 0;
    ddr = 0;
else
    r = (1 - T^(-1)*t)^(q+1)*(cos(3*t))^2;
    dr = -(cos(3*t)*(1 - t/T)^q*(cos(3*t) + q*cos(3*t) - 6*t*sin(3*t) + 6*T*sin(3*t)))/T;
    ddr = 18*sin(3*t)^2*(1 - t/T)^(q + 1) - 18*cos(3*t)^2*(1 - t/T)^(q + 1) + (q*cos(3*t)^2*(q + 1)*(1 - t/T)^(q - 1))/T^2 + (12*cos(3*t)*sin(3*t)*(q + 1)*(1 - t/T)^q)/T;
end
psi = (psi0 - psiinf)*r + psiinf;
dpsi = (psi0 - psiinf)*dr;
ddpsi = (psi0 - psiinf)*ddr;

== matlab function isubsystem_main/Subsystem1/reduced-order dynamic gain observer/MATLAB Function ==
  data: lambda2 input; u input; dlambda2 output; yF input; k2 input; L input; dL input; x2_e output
function [dlambda2,x2_e]= fcn(lambda2,u,yF,k2,L,dL)
%#codegen

x2_e = lambda2 + k2*L*yF;
f1_yF = yF;f2_e = yF*x2_e;
dlambda2 = u + f2_e - k2*L*(x2_e + f1_yF)-k2*dL*yF;

== matlab function isubsystem_main/Subsystem1/reduced-order dynamic gain observer/Subsystem/MATLAB Function2 ==
  data: L input; yF input; dL output; sigma input; theta input; K input; P input; lP input; epsilon1 input; epsilon2 input; epsilon10 input; epsilon20 input; vartheta input
function dL = fcn(L,yF,sigma,theta,K,P,lP,epsilon1,epsilon2,epsilon10,epsilon20,vartheta)
%#codegen

hphou = 1 + 2*(yF)^2 + 2*(vartheta)^2;
a = (-theta + K)/sigma;
b = (norm(P,2)*epsilon1^2)/(lP*sigma) + ((2*epsilon10^2)^(-1)+(2*epsilon20^2)^(-1))/(lP*sigma);
c = (2*(2 + epsilon2^2)*norm(P,2)*(hphou)/(lP*sigma));
%dL = L/sigma*(-theta*L + norm(P,2)*epsilon1^2/lP + ((2*epsilon10^2)^(-1)+(2*epsilon20^2)^(-1))/lP + norm(P,2)*(epsilon2^4 + phou^2)/(lP*epsilon2^2) + K*L);
dL = a*L^2 + b*L + c*L;

== matlab function isubsystem_main/Event-Triggered1/MATLAB Function ==
  data: miu input; E_out output; miu_tk input; eta output; triger output
function [E_out,eta, triger]= fcn(miu,miu_tk)
%#codegen
E_miu = miu_tk;
eta = miu - E_miu;
l1 = 0.2;l2 = 1.5;
triger = (abs(eta)>= l1*abs(E_miu)+l2).*1;
if abs(eta)>= l1*abs(E_miu)+l2
    E_out = miu;
else
    E_out = miu_tk;
end

== matlab function isubsystem_main/Hysteretic Quantizer1/MATLAB Function ==
  data: miu input; Q_miu output; Output_t input; dmiu input
function Q_miu = fcn(miu,Output_t,dmiu)
%#codegen
i = (1:1:100)';
delta = 0.5;miu_min = 0.05;
la = 1 - delta;lb = 1 + delta;lc = la/lb;
miu_i = lc.^(1-i).*miu_min;

if dmiu < 0
    A = (((abs(miu)<=(miu_i/la))*1).*((abs(miu)>(miu_i/lb))*1))';
    miui = A*miu_i;
    if abs(miu) >= 0 && abs(miu) < miu_min/lb
        Output = 0;
    else
        if abs(miu) <= miui && abs(miu) > miui/lb
            Output = miui*sign(miu);
        else
            Output = miui*lb*sign(miu);
        end
    end
elseif dmiu > 0
    A = (((abs(miu)<=(miu_i*lb/la))*1).*((abs(miu)>(miu_i))*1))';
    miui = A*miu_i;
    if abs(miu) >= miu_min/lb && abs(miu) < miu_min
        Output = 0;
    else
        if abs(miu) <= miui/la && abs(miu) > miui
            Output = miui*sign(miu);
        else
            Output = miui*lb*sign(miu);
        end
    end
else
    Output = Output_t;
end

Q_miu = Output;

== matlab function isubsystem_main/Event-Triggered2/MATLAB Function ==
  data: miu input; E_out output; miu_tk input; eta output; triger output
function [E_out,eta, triger]= fcn(miu,miu_tk)
%#codegen
E_miu = miu_tk;
eta = miu - E_miu;
l1 = 0.2;l2 = 1.5;
triger = (abs(eta)>= l1*abs(E_miu)+l2).*1;
if abs(eta)>= l1*abs(E_miu)+l2
    E_out = miu;
else
    E_out = miu_tk;
end

== matlab function isubsystem_main/Hysteretic Quantizer2/MATLAB Function ==
  data: miu input; Q_miu output; Output_t input; dmiu input
function Q_miu = fcn(miu,Output_t,dmiu)
%#codegen
i = (1:1:100)';
delta = 0.5;miu_min = 0.05;
la = 1 - delta;lb = 1 + delta;lc = la/lb;
miu_i = lc.^(1-i).*miu_min;

if dmiu < 0
    A = (((abs(miu)<=(miu_i/la))*1).*((abs(miu)>(miu_i/lb))*1))';
    miui = A*miu_i;
    if abs(miu) >= 0 && abs(miu) < miu_min/lb
        Output = 0;
    else
        if abs(miu) <= miui && abs(miu) > miui/lb
            Output = miui*sign(miu);
        else
            Output = miui*lb*sign(miu);
        end
    end
elseif dmiu > 0
    A = (((abs(miu)<=(miu_i*lb/la))*1).*((abs(miu)>(miu_i))*1))';
    miui = A*miu_i;
    if abs(miu) >= miu_min/lb && abs(miu) < miu_min
        Output = 0;
    else
        if abs(miu) <= miui/la && abs(miu) > miui
            Output = miui*sign(miu);
        else
            Output = miui*lb*sign(miu);
        end
    end
else
    Output = Output_t;
end

Q_miu = Output;

== matlab function isubsystem_main/Subsystem2/Controller1/Subsystem/MATLAB Function1 ==
  data: yF input; dalpha1_dt output; psi input; dpsi input; ddpsi input; L input; W input; Xi input; k2 input; b_low input; b_high input; li input; eta0 input; sigma input; gamma1 input; epsilon10 input; epsilon11 input; epsilon12 input; epsilon13 input; epsilon14 input; epsilon15 input; dalpha1_dW output; dalpha1_dL output; dalpha1_dyF output
function [dalpha1_dt,dalpha1_dW,dalpha1_dL,dalpha1_dyF]= fcn(yF,psi,dpsi,ddpsi,L,W,Xi,k2,b_low,b_high,li,eta0,sigma,gamma1,epsilon10,epsilon11,epsilon12,epsilon13,epsilon14,epsilon15)
%#codegen
dalpha1_dt = (yF*dpsi*(li^2 + yF^2)*(eta0 + 2*gamma1))/(2*li^2*psi^2) - (2*yF^3*dpsi*(b_high - yF/(psi*(li^2 + yF^2)^(1/2)))*(b_low + yF/(psi*(li^2 + yF^2)^(1/2)))*((li^4*(b_high*b_low + yF^2/(psi^2*(li^2 + yF^2)))^2*(epsilon11^2 + epsilon12^2 + epsilon13^2 + epsilon15^2))/(2*(li^2 + yF^2)^3*(b_high - yF/(psi*(li^2 + yF^2)^(1/2)))^4*(b_low + yF/(psi*(li^2 + yF^2)^(1/2)))^4) + (L^(2*sigma)*epsilon10^2*li^4*(b_high*b_low + yF^2/(psi^2*(li^2 + yF^2)))^2)/(2*(li^2 + yF^2)^3*(b_high - yF/(psi*(li^2 + yF^2)^(1/2)))^4*(b_low + yF/(psi*(li^2 + yF^2)^(1/2)))^4) + (epsilon14^2*yF^2*dpsi^2*(b_high*b_low + yF^2/(psi^2*(li^2 + yF^2)))^2)/(2*psi^4*(li^2 + yF^2)*(b_high - yF/(psi*(li^2 + yF^2)^(1/2)))^4*(b_low + yF/(psi*(li^2 + yF^2)^(1/2)))^4)))/(li^2*psi^4*(b_high*b_low + yF^2/(psi^2*(li^2 + yF^2)))^2) + (yF*(li^2 + yF^2)*(b_high - yF/(psi*(li^2 + yF^2)^(1/2)))*(b_low + yF/(psi*(li^2 + yF^2)^(1/2)))*((2*epsilon14^2*yF^2*dpsi*dpsi^2*(b_high*b_low + yF^2/(psi^2*(li^2 + yF^2)))^2)/(psi^5*(li^2 + yF^2)*(b_high - yF/(psi*(li^2 + yF^2)^(1/2)))^4*(b_low + yF/(psi*(li^2 + yF^2)^(1/2)))^4) - (2*epsilon14^2*yF^3*dpsi*dpsi^2*(b_high*b_low + yF^2/(psi^2*(li^2 + yF^2)))^2)/(psi^6*(li^2 + yF^2)^(3/2)*(b_high - yF/(psi*(li^2 + yF^2)^(1/2)))^4*(b_low + yF/(psi*(li^2 + yF^2)^(1/2)))^5) + (2*epsilon14^2*yF^3*dpsi*dpsi^2*(b_high*b_low + yF^2/(psi^2*(li^2 + yF^2)))^2)/(psi^6*(li^2 + yF^2)^(3/2)*(b_high - yF/(psi*(li^2 + yF^2)^(1/2)))^5*(b_low + yF/(psi*(li^2 + yF^2)^(1/2)))^4) - (epsilon14^2*yF^2*ddpsi*dpsi*(b_high*b_low + yF^2/(psi^2*(li^2 + yF^2)))^2)/(psi^4*(li^2 + yF^2)*(b_high - yF/(psi*(li^2 + yF^2)^(1/2)))^4*(b_low + yF/(psi*(li^2 + yF^2)^(1/2)))^4) + (2*epsilon14^2*yF^4*dpsi*dpsi^2*(b_high*b_low + yF^2/(psi^2*(li^2 + yF^2))))/(psi^7*(li^2 + yF^2)^2*(b_high - yF/(psi*(li^2 + yF^2)^(1/2)))^4*(b_low + yF/(psi*(li^2 + yF^2)^(1/2)))^4) + (2*li^4*yF^2*dpsi*(b_high*b_low + yF^2/(psi^2*(li^2 + yF^2)))*(epsilon11^2 + epsilon12^2 + epsilon13^2 + epsilon15^2))/(psi^3*(li^2 + yF^2)^4*(b_high - yF/(psi*(li^2 + yF^2)^(1/2)))^4*(b_low + yF/(psi*(li^2 + yF^2)^(1/2)))^4) - (2*li^4*yF*dpsi*(b_high*b_low + yF^2/(psi^2*(li^2 + yF^2)))^2*(epsilon11^2 + epsilon12^2 + epsilon13^2 + epsilon15^2))/(psi^2*(li^2 + yF^2)^(7/2)*(b_high - yF/(psi*(li^2 + yF^2)^(1/2)))^4*(b_low + yF/(psi*(li^2 + yF^2)^(1/2)))^5) + (2*li^4*yF*dpsi*(b_high*b_low + yF^2/(psi^2*(li^2 + yF^2)))^2*(epsilon11^2 + epsilon12^2 + epsilon13^2 + epsilon15^2))/(psi^2*(li^2 + yF^2)^(7/2)*(b_high - yF/(psi*(li^2 + yF^2)^(1/2)))^5*(b_low + yF/(psi*(li^2 + yF^2)^(1/2)))^4) + (2*L^(2*sigma)*epsilon10^2*li^4*yF^2*dpsi*(b_high*b_low + yF^2/(psi^2*(li^2 + yF^2))))/(psi^3*(li^2 + yF^2)^4*(b_high - yF/(psi*(li^2 + yF^2)^(1/2)))^4*(b_low + yF/(psi*(li^2 + yF^2)^(1/2)))^4) - (2*L^(2*sigma)*epsilon10^2*li^4*yF*dpsi*(b_high*b_low + yF^2/(psi^2*(li^2 + yF^2)))^2)/(psi^2*(li^2 + yF^2)^(7/2)*(b_high - yF/(psi*(li^2 + yF^2)^(1/2)))^4*(b_low + yF/(psi*(li^2 + yF^2)^(1/2)))^5) + (2*L^(2*sigma)*epsilon10^2*li^4*yF*dpsi*(b_high*b_low + yF^2/(psi^2*(li^2 + yF^2)))^2)/(psi^2*(li^2 + yF^2)^(7/2)*(b_high - yF/(psi*(li^2 + yF^2)^(1/2)))^5*(b_low + yF/(psi*(li^2 + yF^2)^(1/2)))^4)))/(li^2*psi*(b_high*b_low + yF^2/(psi^2*(li^2 + yF^2)))) + (yF^2*dpsi*(li^2 + yF^2)^(1/2)*(b_high - yF/(psi*(li^2 + yF^2)^(1/2)))*((li^4*(b_high*b_low + yF^2/(psi^2*(li^2 + yF^2)))^2*(epsilon11^2 + epsilon12^2 + epsilon13^2 + epsilon15^2))/(2*(li^2 + yF^2)^3*(b_high - yF/(psi*(li^2 + yF^2)^(1/2)))^4*(b_low + yF/(psi*(li^2 + yF^2)^(1/2)))^4) + (L^(2*sigma)*epsilon10^2*li^4*(b_high*b_low + yF^2/(psi^2*(li^2 + yF^2)))^2)/(2*(li^2 + yF^2)^3*(b_high - yF/(psi*(li^2 + yF^2)^(1/2)))^4*(b_low + yF/(psi*(li^2 + yF^2)^(1/2)))^4) + (epsilon14^2*yF^2*dpsi^2*(b_high*b_low + yF^2/(psi^2*(li^2 + yF^2)))^2)/(2*psi^4*(li^2 + yF^2)*(b_high - yF/(psi*(li^2 + yF^2)^(1/2)))^4*(b_low + yF/(psi*(li^2 + yF^2)^(1/2)))^4)))/(li^2*psi^3*(b_high*b_low + yF^2/(psi^2*(li^2 + yF^2)))) - (yF^2*dpsi*(li^2 + yF^2)^(1/2)*(b_low + yF/(psi*(li^2 + yF^2)^(1/2)))*((li^4*(b_high*b_low + yF^2/(psi^2*(li^2 + yF^2)))^2*(epsilon11^2 + epsilon12^2 + epsilon13^2 + epsilon15^2))/(2*(li^2 + yF^2)^3*(b_high - yF/(psi*(li^2 + yF^2)^(1/2)))^4*(b_low + yF/(psi*(li^2 + yF^2)^(1/2)))^4) + (L^(2*sigma)*epsilon10^2*li^4*(b_high*b_low + yF^2/(psi^2*(li^2 + yF^2)))^2)/(2*(li^2 + yF^2)^3*(b_high - yF/(psi*(li^2 + yF^2)^(1/2)))^4*(b_low + yF/(psi*(li^2 + yF^2)^(1/2)))^4) + (epsilon14^2*yF^2*dpsi^2*(b_high*b_low + yF^2/(psi^2*(li^2 + yF^2)))^2)/(2*psi^4*(li^2 + yF^2)*(b_high - yF/(psi*(li^2 + yF^2)^(1/2)))^4*(b_low + yF/(psi*(li^2 + yF^2)^(1/2)))^4)))/(li^2*psi^3*(b_high*b_low + yF^2/(psi^2*(li^2 + yF^2)))) + (yF*dpsi*(li^2 + yF^2)*(b_high - yF/(psi*(li^2 + yF^2)^(1/2)))*(b_low + yF/(psi*(li^2 + yF^2)^(1/2)))*((li^4*(b_high*b_low + yF^2/(psi^2*(li^2 + yF^2)))^2*(epsilon11^2 + epsilon12^2 + epsilon13^2 + epsilon15^2))/(2*(li^2 + yF^2)^3*(b_high - yF/(psi*(li^2 + yF^2)^(1/2)))^4*(b_low + yF/(psi*(li^2 + yF^2)^(1/2)))^4) + (L^(2*sigma)*epsilon10^2*li^4*(b_high*b_low + yF^2/(psi^2*(li^2 + yF^2)))^2)/(2*(li^2 + yF^2)^3*(b_high - yF/(psi*(li^2 + yF^2)^(1/2)))^4*(b_low + yF/(psi*(li^2 + yF^2)^(1/2)))^4) + (epsilon14^2*yF^2*dpsi^2*(b_high*b_low + yF^2/(psi^2*(li^2 + yF^2)))^2)/(2*psi^4*(li^2 + yF^2)*(b_high - yF/(psi*(li^2 + yF^2)^(1/2)))^4*(b_low + yF/(psi*(li^2 + yF^2)^(1/2)))^4)))/(li^2*psi^2*(b_high*b_low + yF^2/(psi^2*(li^2 + yF^2)))) - (yF*dpsi*(li^2 + yF^2)*(b_high - yF/(psi*(li^2 + yF^2)^(1/2)))*(b_low + yF/(psi*(li^2 + yF^2)^(1/2)))^2*(eta0*yF*psi*(li^2 + yF^2)^(1/2) - 2*W'*Xi*yF^2 + 2*gamma1*yF*psi*(li^2 + yF^2)^(1/2) + 2*W'*Xi*b_high*yF*psi*(li^2 + yF^2)^(1/2) - 2*W'*Xi*b_low*yF*psi*(li^2 + yF^2)^(1/2) + 2*W'*Xi*b_high*b_low*li^2*psi^2 + 2*W'*Xi*b_high*b_low*yF^2*psi^2))/(li^2*psi^2*(b_high*b_low + yF^2/(psi^2*(li^2 + yF^2)))*(b_high*b_low*li^2*psi^2 - yF^2 + b_high*b_low*yF^2*psi^2 + b_high*yF*psi*(li^2 + yF^2)^(1/2) - b_low*yF*psi*(li^2 + yF^2)^(1/2))) + (yF*dpsi*(li^2 + yF^2)*(b_high - yF/(psi*(li^2 + yF^2)^(1/2)))^2*(b_low + yF/(psi*(li^2 + yF^2)^(1/2)))*(eta0*yF*psi*(li^2 + yF^2)^(1/2) - 2*W'*Xi*yF^2 + 2*gamma1*yF*psi*(li^2 + yF^2)^(1/2) + 2*W'*Xi*b_high*yF*psi*(li^2 + yF^2)^(1/2) - 2*W'*Xi*b_low*yF*psi*(li^2 + yF^2)^(1/2) + 2*W'*Xi*b_high*b_low*li^2*psi^2 + 2*W'*Xi*b_high*b_low*yF^2*psi^2))/(li^2*psi^2*(b_high*b_low + yF^2/(psi^2*(li^2 + yF^2)))*(b_high*b_low*li^2*psi^2 - yF^2 + b_high*b_low*yF^2*psi^2 + b_high*yF*psi*(li^2 + yF^2)^(1/2) - b_low*yF*psi*(li^2 + yF^2)^(1/2))) - (yF^2*dpsi*(li^2 + yF^2)^(1/2)*(b_high - yF/(psi*(li^2 + yF^2)^(1/2)))^2*(b_low + yF/(psi*(li^2 + yF^2)^(1/2)))^2*(eta0*yF*psi*(li^2 + yF^2)^(1/2) - 2*W'*Xi*yF^2 + 2*gamma1*yF*psi*(li^2 + yF^2)^(1/2) + 2*W'*Xi*b_high*yF*psi*(li^2 + yF^2)^(1/2) - 2*W'*Xi*b_low*yF*psi*(li^2 + yF^2)^(1/2) + 2*W'*Xi*b_high*b_low*li^2*psi^2 + 2*W'*Xi*b_high*b_low*yF^2*psi^2))/(li^2*psi^3*(b_high*b_low + yF^2/(psi^2*(li^2 + yF^2)))^2*(b_high*b_low*li^2*psi^2 - yF^2 + b_high*b_low*yF^2*psi^2 + b_high*yF*psi*(li^2 + yF^2)^(1/2) - b_low*yF*psi*(li^2 + yF^2)^(1/2)));
dalpha1_dW = -(Xi*(li^2 + yF^2)^(3/2)*(b_high - yF/(psi*(li^2 + yF^2)^(1/2)))^2*(b_low + yF/(psi*(li^2 + yF^2)^(1/2)))^2)/(li^2*(b_high*b_low + yF^2/(psi^2*(li^2 + yF^2)))); 
dalpha1_dL = - k2*yF - (L^(2*sigma - 1)*epsilon10^2*li^2*sigma*yF*(b_high*b_low + yF^2/(psi^2*(li^2 + yF^2))))/(psi*(li^2 + yF^2)^2*(b_high - yF/(psi*(li^2 + yF^2)^(1/2)))^3*(b_low + yF/(psi*(li^2 + yF^2)^(1/2)))^3);
dalpha1_dyF = (b_high - yF/(psi*(li^2 + yF^2)^(1/2)))*(b_low + yF/(psi*(li^2 + yF^2)^(1/2)))^2*(eta0*yF*psi*(li^2 + yF^2)^(1/2) - 2*W'*Xi*yF^2 + 2*gamma1*yF*psi*(li^2 + yF^2)^(1/2) + 2*W'*Xi*b_high*yF*psi*(li^2 + yF^2)^(1/2) - 2*W'*Xi*b_low*yF*psi*(li^2 + yF^2)^(1/2) + 2*W'*Xi*b_high*b_low*li^2*psi^2 + 2*W'*Xi*b_high*b_low*yF^2*psi^2);

== matlab function isubsystem_main/Subsystem2/Controller1/Subsystem1/MATLAB Function2 ==
  data: dalpha1_dt input; dalpha1_dW input; dalpha1_dL input; dalpha1_dyF input; alpha1 input; yF input; lambda2 input; alpha2 output; dW input; dL input; L input; k2 input; gamma2 input; sigma input; epsilon20 input; epsilon11 input; epsilon22 input; epsilon23 input; epsilon24 input; epsilon25 input; z2 output
function [alpha2,z2] = fcn(dalpha1_dt,dalpha1_dW,dalpha1_dL,dalpha1_dyF,alpha1,yF,lambda2,dW,dL,L,k2,gamma2,sigma,epsilon20,epsilon11,epsilon22,epsilon23,epsilon24,epsilon25)
%#codegen

z2 = lambda2 - alpha1;
x2_e = lambda2 + k2*L*yF;
f1_yF = yF;f2_e = yF*x2_e;
alpha2 = f2_e - k2*L*(x2_e + f1_yF) - k2*dL*yF - dW'*dalpha1_dW - dalpha1_dL*dL - dalpha1_dt - dalpha1_dyF*(x2_e + f1_yF) + 0.5*z2*dalpha1_dyF^2*((epsilon20*L^sigma)^2 + epsilon22^2 + epsilon23^2 + epsilon25^2) + epsilon24^2*z2 + z2/(2*epsilon11^2) + gamma2*z2;

== matlab function isubsystem_main/Subsystem2/Controller1/Subsystem2/MATLAB Function ==
  data: alpha2 input; v output; alpha1 input; lambda2 input; l1 input; l2 input; w input
function v = fcn(alpha2,alpha1,lambda2,l1,l2,w)
%#codegen
delta = 0.5;la = 1 - delta;
z2 = lambda2 - alpha1;
zetad = sqrt(z2^2*alpha2^2 + w^2);
%zetal = sqrt(z2^2*l2^2 + (1 - l1)^2*w^2);
zetal = sqrt(z2^2*l2^2 + w^2);
%v = -(1 + l1)*z2*(alpha2^2/zetad + l2^2/((1 - l1)*zetal));
v = -la^(-1)*z2*(alpha2^2/zetad + l2^2/(zetal));

== matlab function isubsystem_main/Subsystem2/Controller1/Subsystem3/MATLAB Function1 ==
  data: yF input; alpha1 output; psi input; dpsi input; L input; W input; Xi input; k2 input; b_low input; b_high input; li input; eta0 input; sigma input; gamma1 input; epsilon10 input; epsilon11 input; epsilon12 input; epsilon13 input; epsilon14 input; epsilon15 input; z1 output
function [alpha1,z1]= fcn(yF,psi,dpsi,L,W,Xi,k2,b_low,b_high,li,eta0,sigma,gamma1,epsilon10,epsilon11,epsilon12,epsilon13,epsilon14,epsilon15)
%#codegen
f1_yF = yF;
X = yF/(psi*sqrt(yF^2 + li^2));
z1 = X/((b_low + X)*(b_high - X));
h1 = li^2*(b_low*b_high + X^2)/((b_low+X)^2*(b_high-X)^2*(yF^2 + li^2)^(3/2));
h2 = -dpsi*yF*(b_low*b_high + X^2)/(psi^2*(b_low+X)^2*(b_high-X)^2*sqrt(yF^2 + li^2));
alpha1 = - k2*L*yF - f1_yF - h1^(-1)*(W'*Xi + gamma1*z1 + eta0/2*z1)-z1*h1^(-1)*(0.5*(epsilon10*h1*L^sigma)^2 + 0.5*h1^2*(epsilon11^2 + epsilon12^2 + epsilon13^2 + epsilon15^2) + 0.5*(epsilon14*h2)^2);

== matlab function isubsystem_main/Subsystem2/Fuzzy/MATLAB Function ==
  data: W input; yF input; Xi output; dW output; z1 input; Psi input; eta1 input
function [Xi,dW]= fcn(W,yF,z1,Psi,eta1)
%#codegen

Xi = [exp(-0.5*(yF - 8)^2);exp(-0.5*(yF - 4)^2);exp(-0.5*yF^2);exp(-0.5*(yF + 4)^2);exp(-0.5*(yF + 8)^2)];
dW = Psi*z1*Xi - eta1*Psi*W;

== matlab function isubsystem_main/Subsystem2/PPF /MATLAB Function ==
  data: psi0 input; psi output; dpsi output; psiinf input; T input; q input; t input; ddpsi output
function [psi,dpsi,ddpsi]= fcn(psi0,psiinf,T,q,t)
%#codegen
if t >= T
    r = 0;
    dr = 0;
    ddr = 0;
else
    r = (1 - T^(-1)*t)^(q+1)*(cos(3*t))^2;
    dr = -(cos(3*t)*(1 - t/T)^q*(cos(3*t) + q*cos(3*t) - 6*t*sin(3*t) + 6*T*sin(3*t)))/T;
    ddr = 18*sin(3*t)^2*(1 - t/T)^(q + 1) - 18*cos(3*t)^2*(1 - t/T)^(q + 1) + (q*cos(3*t)^2*(q + 1)*(1 - t/T)^(q - 1))/T^2 + (12*cos(3*t)*sin(3*t)*(q + 1)*(1 - t/T)^q)/T;
end
psi = (psi0 - psiinf)*r + psiinf;
dpsi = (psi0 - psiinf)*dr;
ddpsi = (psi0 - psiinf)*ddr;

== matlab function isubsystem_main/Subsystem2/reduced-order dynamic gain observer/MATLAB Function ==
  data: lambda2 input; u input; dlambda2 output; yF input; k2 input; L input; dL input; x2_e output
function [dlambda2,x2_e]= fcn(lambda2,u,yF,k2,L,dL)
%#codegen

x2_e = lambda2 + k2*L*yF;
f1_yF = yF;f2_e = yF*x2_e;
dlambda2 = u + f2_e - k2*L*(x2_e + f1_yF)-k2*dL*yF;

== matlab function isubsystem_main/Subsystem2/reduced-order dynamic gain observer/Subsystem/MATLAB Function2 ==
  data: L input; yF input; dL output; sigma input; theta input; K input; P input; lP input; epsilon1 input; epsilon2 input; epsilon10 input; epsilon20 input; vartheta input
function dL = fcn(L,yF,sigma,theta,K,P,lP,epsilon1,epsilon2,epsilon10,epsilon20,vartheta)
%#codegen

hphou = 1 + 2*(yF)^2 + 2*(vartheta)^2;
a = (-theta + K)/sigma;
b = (norm(P,2)*epsilon1^2)/(lP*sigma) + ((2*epsilon10^2)^(-1)+(2*epsilon20^2)^(-1))/(lP*sigma);
c = (2*(2 + epsilon2^2)*norm(P,2)*(hphou)/(lP*sigma));
%dL = L/sigma*(-theta*L + norm(P,2)*epsilon1^2/lP + ((2*epsilon10^2)^(-1)+(2*epsilon20^2)^(-1))/lP + norm(P,2)*(epsilon2^4 + phou^2)/(lP*epsilon2^2) + K*L);
dL = a*L^2 + b*L + c*L;

== matlab function isubsystem_main/PPF 1/MATLAB Function ==
  data: psi0 input; P_up output; P_down output; psiinf input; T input; q input; t input
function [P_up,P_down]= fcn(psi0,psiinf,T,q,t)
%#codegen
if t >= T
    r = 0;
    dr = 0;
    ddr = 0;
else
    r = (1 - T^(-1)*t)^(q+1)*(cos(3*t))^2;
    dr = -(cos(3*t)*(1 - t/T)^q*(cos(3*t) + q*cos(3*t) - 6*t*sin(3*t) + 6*T*sin(3*t)))/T;
    ddr = 18*sin(3*t)^2*(1 - t/T)^(q + 1) - 18*cos(3*t)^2*(1 - t/T)^(q + 1) + (q*cos(3*t)^2*(q + 1)*(1 - t/T)^(q - 1))/T^2 + (12*cos(3*t)*sin(3*t)*(q + 1)*(1 - t/T)^q)/T;
end
psi = (psi0 - psiinf)*r + psiinf;
dpsi = (psi0 - psiinf)*dr;
ddpsi = (psi0 - psiinf)*ddr;

P_up = psi/sqrt(1 - psi^2);
P_down = -psi/sqrt(1 - psi^2);
